simulink model "final_steady_24a"  (R2025a)
settings: Solver=ode15s  StartTime=0.0  StopTime=14000  RelTol=1e-3
undefined symbols (not defined in the file): bp_er, bp_mf, bp_speed, Cp_rad, epsilon, ETAT_table, m_ratio_bp, PR_table, speed_bp, table_eff, table_mf, theta
(part 1 of 2)
settings Model: Creator=HeY  LastModifiedBy=ikunsredemptionmac
settings DataIOCC: InitialState=xfinal  SaveFinalState=on  SaveOperatingPoint=on

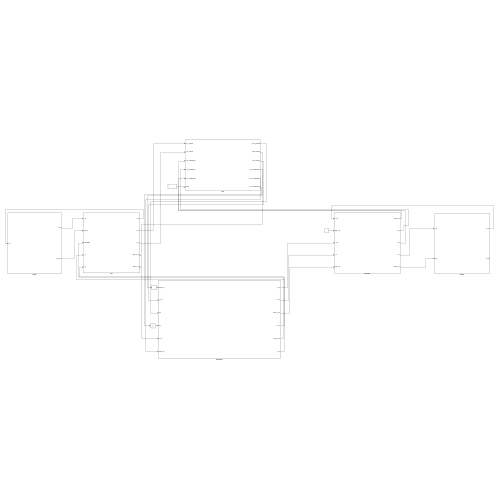
[thumbnail: Simulink's stored preview of the top-level diagram]
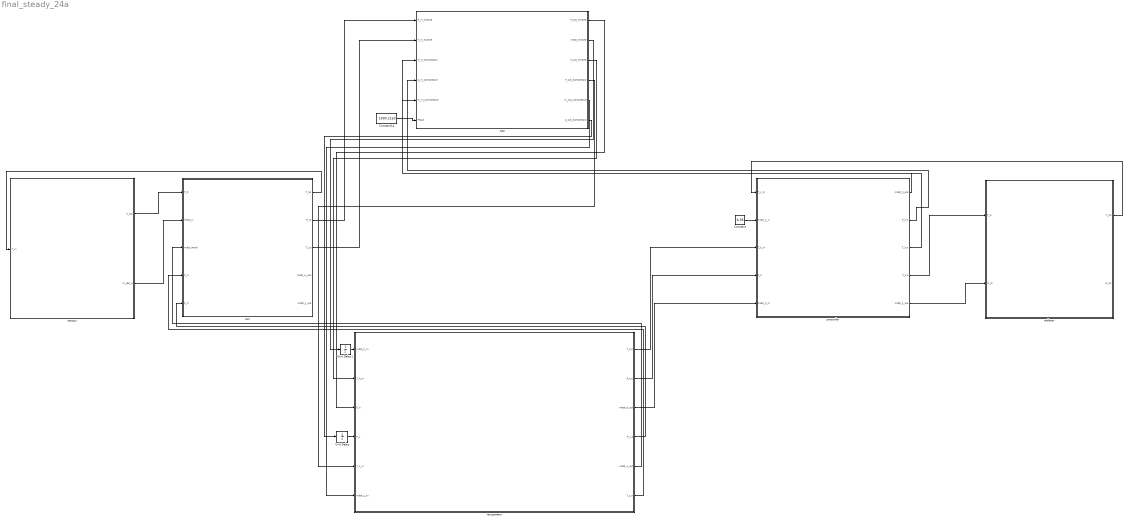
== system final_steady_24a ==
  Constant : Constant  Value=6.95
  Constant14 : Constant  Value=1000.21e3
  IHX : Subsystem
  TAC : Subsystem
  Unit Delay : UnitDelay  InitialCondition=1.551e6  SampleTime=-1  HasFrameUpgradeWarning=on
  Unit Delay1 : UnitDelay  InitialCondition=11.982029  SampleTime=-1  HasFrameUpgradeWarning=on
  precooler : Subsystem
  reactor : Subsystem
  recuperator : Subsystem
  rediator : Subsystem
  wires:
  reactor/1(T_out) -> IHX/1(T_hi)
  IHX/1(T_ho) -> reactor/1(T_in)
  reactor/2(m_dot_Li) -> IHX/2(mdot_Li)
  recuperator/6(T_c,o) -> IHX/4(T_ci)
  recuperator/4(P_c,o) -> IHX/5(P_ci)
  IHX/2(P_co) -> TAC/1(P_in_Turbine)
  IHX/3(T_co) -> TAC/2(T_in_Turbine)
  recuperator/5(mdot_c_out) -> IHX/3(mdot_HeXe)
  recuperator/3(mdot_h_out) -> precooler/5(mdot_h_in)
  recuperator/2(P_h,o) -> precooler/4(P_h)
  recuperator/1(T_h,o) -> precooler/3(T_h_in)
  Constant/1 -> precooler/2(mdot_c_in)
  precooler/3(T_h,o) -> TAC/3(T_in_Compressor)
  precooler/4(T_c,o) -> rediator/1(T_hi)
  precooler/5(mdot_c_out) -> rediator/2(m_hi)
  rediator/1(T_ho) -> precooler/1(T_c_in)
  precooler/1(mdot_h_out) -> TAC/5(m_in_Compressor)
  precooler/2(P_h,o) -> TAC/4(p_in_Compressor)
  Unit Delay/1 -> recuperator/4(P_c)
  TAC/2(mdot_Turbine) -> Unit Delay1/1
  TAC/3(T_out_Turbine) -> recuperator/2(T_h_in)
  TAC/4(T_out_Compressor) -> recuperator/5(T_c_in)
  TAC/5(m_out_Compressor) -> recuperator/6(mdot_c_in)
  TAC/6(p_out_Compressor) -> Unit Delay/1
  Constant14/1 -> TAC/6(Pload)
  TAC/1(P_out_Turbine) -> recuperator/3(P_h)
  Unit Delay1/1 -> recuperator/1(mdot_h_in)

== system final_steady_24a/IHX ==
  T_hi : Inport
  mdot_Li : Inport  Port=2
  mdot_HeXe : Inport  Port=3
  T_ci : Inport  Port=4
  P_ci : Inport  Port=5
  IHX_region_1 : Subsystem
  IHX_region_2 : Subsystem
  Scope : Scope
      settings: ActiveDisplayYMinimum=1527.0598  ActiveDisplayYMaximum=1529.6517
  Scope1 : Scope
      settings: ActiveDisplayYMinimum=1413.1189  ActiveDisplayYMaximum=1443.3824
  T_ho : Outport
  P_co : Outport  Port=2
  T_co : Outport  Port=3
  mdot_Li_out : Outport  Port=4
  mdot_c_out : Outport  Port=5
  wires:
  mdot_Li/1 -> IHX_region_1/3(mdot_Li_in)
  P_ci/1 -> IHX_region_1/2(P_HeXe_in)
  IHX_region_1/4(mdot_HeXe_out) -> mdot_c_out/1
  IHX_region_1/1(T_Li_out) -> IHX_region_2/1(T_Li_in)
  IHX_region_1/5(T_HeXe_out) -> Scope/1, T_co/1
  IHX_region_1/2(P_HeXe_out) -> IHX_region_2/2(P_HeXe_in)
  IHX_region_2/2(P_HeXe_out) -> P_co/1
  T_hi/1 -> IHX_region_1/1(T_Li_in)
  mdot_HeXe/1 -> IHX_region_2/4(mdot_HeXe_in)
  IHX_region_2/3(mdot_Li_out) -> mdot_Li_out/1
  IHX_region_2/1(T_Li_out) -> Scope1/1, T_ho/1
  IHX_region_2/4(mdot_HeXe_out) -> IHX_region_1/4(mdot_HeXe_in)
  IHX_region_2/5(T_HeXe_out) -> IHX_region_1/5(T_HeXe_in)
  T_ci/1 -> IHX_region_2/5(T_HeXe_in)
  IHX_region_1/3(mdot_Li_out) -> IHX_region_2/3(mdot_Li_in)

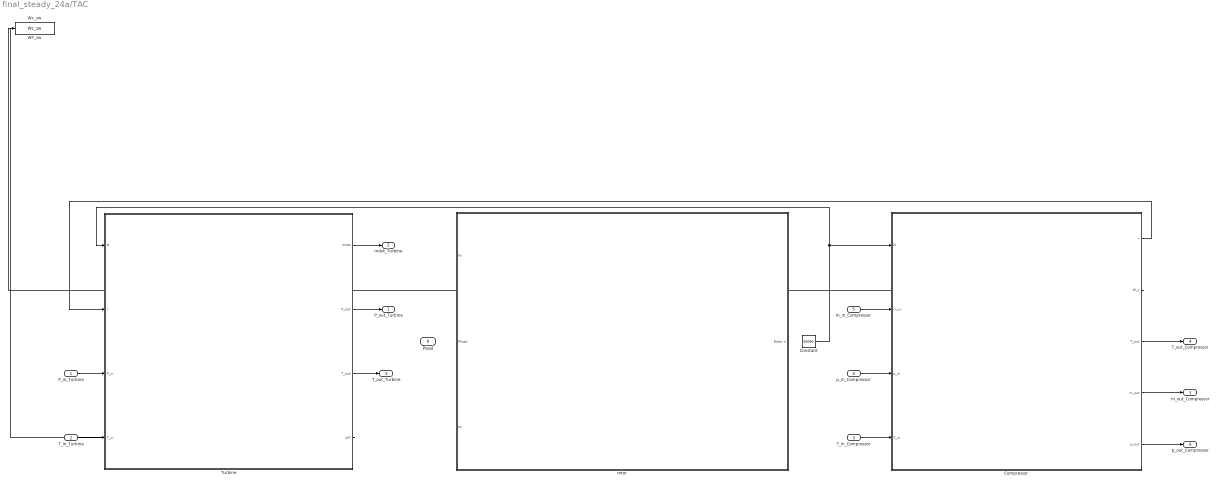
== system final_steady_24a/TAC ==
  P_in_Turbine : Inport
  T_in_Turbine : Inport  Port=2
  T_in_Compressor : Inport  Port=3
  p_in_Compressor : Inport  Port=4
  m_in_Compressor : Inport  Port=5
  Pload : Inport  Port=6
  Compressor : Subsystem
  Constant : Constant  Value=55090
  Turbine : Subsystem
  WT_sw : ToWorkspace  VariableName=WT_sw  SaveFormat=Timeseries  SampleTime=-1
  Wc_sw : ToWorkspace  VariableName=Wc_sw  SaveFormat=Timeseries  SampleTime=-1
  rotor : Subsystem
  P_out_Turbine : Outport
  mdot_Turbine : Outport  Port=2
  T_out_Turbine : Outport  Port=3
  T_out_Compressor : Outport  Port=4
  m_out_Compressor : Outport  Port=5
  p_out_Compressor : Outport  Port=6
  wires:
  Compressor/1(r) -> Turbine/2(r)
  P_in_Turbine/1 -> Turbine/3(P_in)
  T_in_Turbine/1 -> Turbine/4(T_in)
  Turbine/1(mdot) -> mdot_Turbine/1
  Turbine/2(P_out) -> P_out_Turbine/1
  Turbine/3(T_out) -> T_out_Turbine/1
  m_in_Compressor/1 -> Compressor/2(m_in)
  p_in_Compressor/1 -> Compressor/3(p_in)
  T_in_Compressor/1 -> Compressor/4(T_in)
  Compressor/3(T_out) -> T_out_Compressor/1
  Compressor/4(m_out) -> m_out_Compressor/1
  Compressor/5(p_out) -> p_out_Compressor/1
  Constant/1 -> Turbine/1(N), Compressor/1(N)
  Turbine/4(WT) -> WT_sw/1
  Compressor/2(W_c) -> Wc_sw/1

== system final_steady_24a/precooler ==
  T_c_in : Inport
  mdot_c_in : Inport  Port=2
  T_h_in : Inport  Port=3
  P_h : Inport  Port=4
  mdot_h_in : Inport  Port=5
  Scope1 : Scope
      settings: ActiveDisplayYMinimum=380.7971  ActiveDisplayYMaximum=621.9029
  precooler_1 : Subsystem
  precooler_2 : Subsystem
  mdot_h_out : Outport
  P_h,o : Outport  Port=2
  T_h,o : Outport  Port=3
  T_c,o : Outport  Port=4
  mdot_c_out : Outport  Port=5
  wires:
  precooler_1/5(T_c,o) -> T_c,o/1
  mdot_c_in/1 -> precooler_2/4(mdot_c_in)
  P_h/1 -> precooler_1/2(P_h)
  precooler_1/2(P_h,o) -> precooler_2/2(P_h)
  precooler_1/4(mdot_c_out) -> mdot_c_out/1
  precooler_2/5(T_c,o) -> precooler_1/5(T_c_in)
  precooler_1/3(mdot_h_out) -> precooler_2/3(mdot_h_in)
  precooler_1/1(T_h,o) -> precooler_2/1(T_h_in)
  mdot_h_in/1 -> precooler_1/3(mdot_h_in)
  precooler_2/2(P_h,o) -> P_h,o/1
  T_h_in/1 -> precooler_1/1(T_h_in)
  precooler_2/4(mdot_c_out) -> precooler_1/4(mdot_c_in)
  T_c_in/1 -> precooler_2/5(T_c_in)
  precooler_2/3(mdot_h_out) -> mdot_h_out/1
  precooler_2/1(T_h,o) -> Scope1/1, T_h,o/1

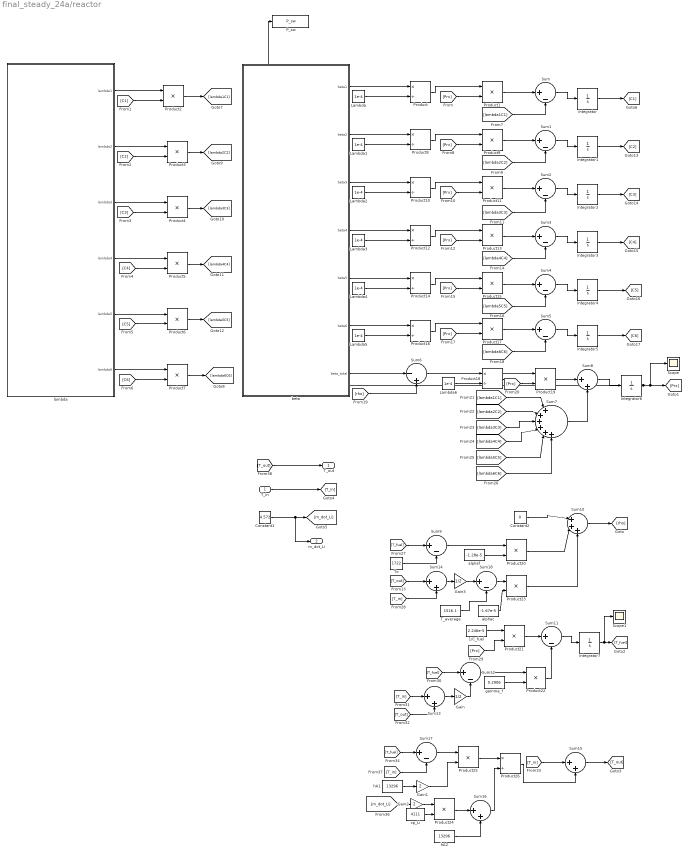
== system final_steady_24a/reactor ==
  T_in : Inport
  1/C_fuel : Constant  Value=2.246e-5
  Constant1 : Constant  Value=4.572
  Constant2 : Constant  Value=0
  Gain : Gain  Gain=1/2
  Gain1 : Gain  Gain=2
  Gain2 : Gain  Gain=2
  Gain3 : Gain  Gain=1/2
  Integrator : Integrator  InitialCondition=509563538.35378009
  Integrator1 : Integrator  InitialCondition=1144297134.5374382
  Integrator2 : Integrator  InitialCondition=278405927.94625711
  Integrator3 : Integrator  InitialCondition=222870449.79609099
  Integrator4 : Integrator  InitialCondition=15570422.720039152
  Integrator5 : Integrator  InitialCondition=1144144.4343794831
  Integrator6 : Integrator  InitialCondition=2660960.9141046703
  Integrator7 : Integrator  InitialCondition=1721.8648882133552
  Lambda{,1..6} (7 alike) : Constant  Value=1e-4
  P_sw : ToWorkspace  VariableName=P_sw  SaveFormat=Timeseries  SampleTime=-1
  Product{,8,10,12,14,16,18,26} (8 alike) : Product  Inputs=*/
  Product{1..7,9,11,13,15,17,19..25} (19 alike) : Product
  Scope : Scope
      settings: ActiveDisplayYMinimum=-1  ActiveDisplayYMaximum=1  DataLoggingVariableName=ScopeData2
  Scope1 : Scope
      settings: ActiveDisplayYMinimum=-1  ActiveDisplayYMaximum=1  DataLoggingVariableName=ScopeData3
  Sum{,1..5,9,11..12,17..18} (11 alike) : Sum  Inputs=|+-
  Sum10 : Sum  Inputs=|+++
  Sum{8,13..16} (5 alike) : Sum  Inputs=|++
  Sum6 : Sum  Inputs=|-+
  Sum7 : Sum  Inputs=|++++++
  T_average : Constant  Value=1516.1
  To : Constant  Value=1722
  alphac : Constant  Value=-1.67e-5
  alphaf : Constant  Value=-1.28e-5
  beta : Subsystem
  cp_Li : Constant  Value=4111
  gamma_f : Constant  Value=0.2906
  hA1 : Constant  Value=13296
  hA2 : Constant  Value=13296
  lambda : Subsystem
  T_out : Outport
  m_dot_Li : Outport  Port=2
  wires:
  Lambda/1 -> Product/2
  beta/1(beta1) -> Product/1
  Product/1 -> Product1/1
  [Prx] -> Product1/2
  Product1/1 -> Sum/1
  [C1] -> Product2/2
  lambda/1(lambda1) -> Product2/1
  lambda/2(lambda2) -> Product3/1
  [C2] -> Product3/2
  lambda/3(lambda3) -> Product4/1
  lambda/4(lambda4) -> Product5/1
  lambda/5(lambda5) -> Product6/1
  lambda/6(lambda6) -> Product7/1
  [C6] -> Product7/2
  [C5] -> Product6/2
  [C4] -> Product5/2
  [C3] -> Product4/2
  Product2/1 -> [lambda1C1]
  Product3/1 -> [lambda2C2]
  Product7/1 -> [lambda6C6]
  Product6/1 -> [lambda5C5]
  Product5/1 -> [lambda4C4]
  Product4/1 -> [lambda3C3]
  [lambda1C1] -> Sum/2
  Sum/1 -> Integrator/1
  Integrator/1 -> [C1]
  Integrator1/1 -> [C2]
  Sum1/1 -> Integrator1/1
  [lambda2C2] -> Sum1/2
  Product9/1 -> Sum1/1
  [Prx] -> Product9/2
  Product8/1 -> Product9/1
  beta/2(beta2) -> Product8/1
  Lambda1/1 -> Product8/2
  Lambda2/1 -> Product10/2
  beta/3(beta3) -> Product10/1
  Product10/1 -> Product11/1
  [Prx] -> Product11/2
  Product11/1 -> Sum2/1
  [lambda3C3] -> Sum2/2
  Sum2/1 -> Integrator2/1
  Integrator2/1 -> [C3]
  Integrator3/1 -> [C4]
  Sum3/1 -> Integrator3/1
  [lambda4C4] -> Sum3/2
  Product13/1 -> Sum3/1
  [Prx] -> Product13/2
  Product12/1 -> Product13/1
  Lambda3/1 -> Product12/2
  beta/4(beta4) -> Product12/1
  beta/5(beta5) -> Product14/1
  Lambda4/1 -> Product14/2
  Product14/1 -> Product15/1
  [Prx] -> Product15/2
  Product15/1 -> Sum4/1
  [lambda5C5] -> Sum4/2
  Sum4/1 -> Integrator4/1
  Integrator4/1 -> [C5]
  Integrator5/1 -> [C6]
  Sum5/1 -> Integrator5/1
  [lambda6C6] -> Sum5/2
  Product17/1 -> Sum5/1
  [Prx] -> Product17/2
  Product16/1 -> Product17/1
  Lambda5/1 -> Product16/2
  beta/6(beta6) -> Product16/1
  beta/7(beta_total) -> Sum6/1
  [rho] -> Sum6/2
  Sum6/1 -> Product18/1
  Lambda6/1 -> Product18/2
  Product18/1 -> Product19/1
  [Prx] -> Product19/2
  [lambda1C1] -> Sum7/1
  [lambda2C2] -> Sum7/2
  [lambda3C3] -> Sum7/3
  [lambda4C4] -> Sum7/4
  [lambda5C5] -> Sum7/5
  [lambda6C6] -> Sum7/6
  Sum7/1 -> Sum8/2
  Product19/1 -> Sum8/1
  Sum8/1 -> Integrator6/1
  Integrator6/1 -> Scope/1, [Prx], P_sw/1
  [T_fuel] -> Sum9/1
  To/1 -> Sum9/2
  Sum9/1 -> Product20/1
  alphaf/1 -> Product20/2
  Product20/1 -> Sum10/2
  Constant2/1 -> Sum10/1
  Sum10/1 -> [rho]
  1/C_fuel/1 -> Product21/1
  [Prx] -> Product21/2
  Product21/1 -> Sum11/1
  [T_fuel] -> Sum12/1
  [T_in] -> Sum13/1
  [T_out] -> Sum13/2
  Sum13/1 -> Gain/1
  Gain/1 -> Sum12/2
  Sum12/1 -> Product22/1
  gamma_f/1 -> Product22/2
  Product22/1 -> Sum11/2
  Sum11/1 -> Integrator7/1
  Integrator7/1 -> Scope1/1, [T_fuel]
  T_in/1 -> [T_in]
  Constant1/1 -> m_dot_Li/1, [m_dot_Li]
  [T_in] -> Sum15/1
  hA1/1 -> Gain1/1
  [m_dot_Li] -> Gain2/1
  Gain2/1 -> Product24/1
  cp_Li/1 -> Product24/2
  Product24/1 -> Sum16/1
  hA2/1 -> Sum16/2
  [T_fuel] -> Sum17/1
  [T_in] -> Sum17/2
  Sum17/1 -> Product25/1
  Gain1/1 -> Product25/2
  Product25/1 -> Product26/1
  Sum16/1 -> Product26/2
  Product26/1 -> Sum15/2
  Sum15/1 -> [T_out]
  [T_out] -> T_out/1
  Product23/1 -> Sum10/3
  alphac/1 -> Product23/2
  [T_out] -> Sum14/1
  [T_in] -> Sum14/2
  Sum14/1 -> Gain3/1
  Gain3/1 -> Sum18/1
  Sum18/1 -> Product23/1
  T_average/1 -> Sum18/2

== system final_steady_24a/recuperator ==
  mdot_h_in : Inport  OutDataTypeStr=double  Unit=kg/s  PortDimensions=1  Interpolate=off
  T_h_in : Inport  Port=2  OutDataTypeStr=double  Unit=K  PortDimensions=1  Interpolate=off
  P_h : Inport  Port=3  OutDataTypeStr=double  Unit=Pa  PortDimensions=1  Interpolate=off
  P_c : Inport  Port=4  OutDataTypeStr=double  Unit=Pa  PortDimensions=1  Interpolate=off
  T_c_in : Inport  Port=5  OutDataTypeStr=double  Unit=K  PortDimensions=1  Interpolate=off
  mdot_c_in : Inport  Port=6  OutDataTypeStr=double  Unit=kg/s  PortDimensions=1  Interpolate=off
  MannRegion_1 : Subsystem
  MannRegion_2 : Subsystem
  T_h,o : Outport  OutDataTypeStr=double  Unit=K  PortDimensions=1
  P_h,o : Outport  Port=2  OutDataTypeStr=double  Unit=Pa  PortDimensions=1
  mdot_h_out : Outport  Port=3  OutDataTypeStr=double  Unit=kg/s  PortDimensions=1
  P_c,o : Outport  Port=4  OutDataTypeStr=double  Unit=Pa  PortDimensions=1
  mdot_c_out : Outport  Port=5  OutDataTypeStr=double  Unit=kg/s  PortDimensions=1
  T_c,o : Outport  Port=6  OutDataTypeStr=double  Unit=K  PortDimensions=1
  wires:
  MannRegion_1/1(mdot_h_out) -> MannRegion_2/1(mdot_h_in)
  MannRegion_2/4(mdot_c_out) -> MannRegion_1/4(mdot_c_in)
  MannRegion_1/3(T_h,o) -> MannRegion_2/3(T_h_in)
  T_h_in/1 -> MannRegion_1/1(T_h_in)
  P_h/1 -> MannRegion_1/3(P_h)
  MannRegion_2/6(P_c,o) -> MannRegion_1/6(P_c)
  MannRegion_1/4(mdot_c_out) -> mdot_c_out/1
  MannRegion_1/6(P_c,o) -> P_c,o/1
  MannRegion_1/2(P_h,o) -> MannRegion_2/2(P_h)
  MannRegion_1/5(T_c,o) -> T_c,o/1
  mdot_h_in/1 -> MannRegion_1/2(mdot_h_in)
  P_c/1 -> MannRegion_2/6(P_c)
  T_c_in/1 -> MannRegion_2/5(T_c_in)
  mdot_c_in/1 -> MannRegion_2/4(mdot_c_in)
  MannRegion_2/2(P_h,o) -> P_h,o/1
  MannRegion_2/3(T_h,o) -> T_h,o/1
  MannRegion_2/1(mdot_h_out) -> mdot_h_out/1
  MannRegion_2/5(T_c,o) -> MannRegion_1/5(T_c_in)

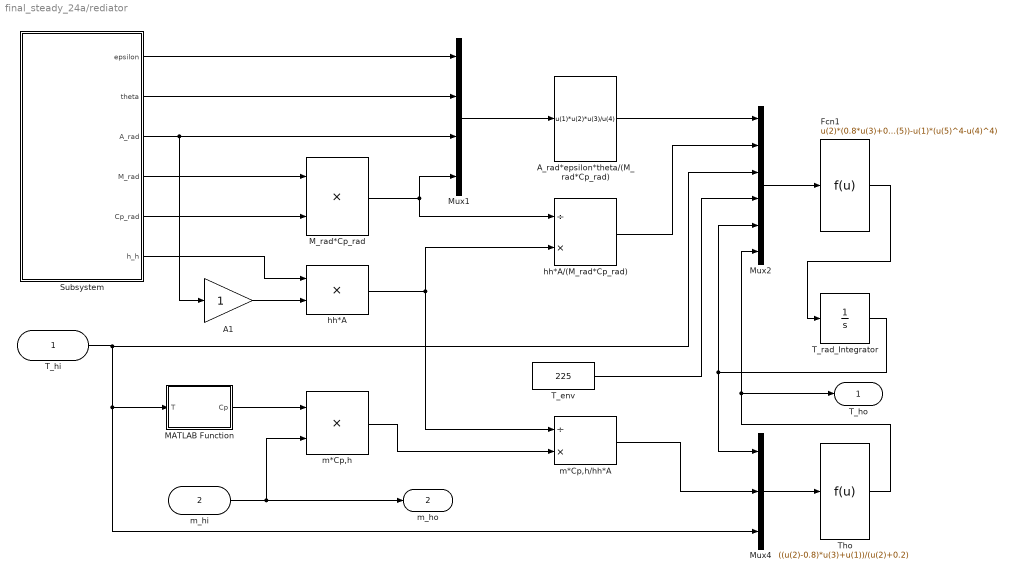
== system final_steady_24a/rediator ==
  T_hi : Inport
  m_hi : Inport  Port=2
  A1 : Gain
  A_rad*epsilon*theta/(M_rad*Cp_rad) : Fcn  Expr=u(1)*u(2)*u(3)/u(4)
  Fcn1 : Fcn  Expr=u(2)*(0.8*u(3)+0.2*u(6)-u(5))-u(1)*(u(5)^4-u(4)^4)
  MATLAB Function : MATLAB Function  TreatAsAtomicUnit=on
  M_rad*Cp_rad : Product
  Mux1 : Mux
  Mux2 : Mux  Inputs=6
  Mux4 : Mux  Inputs=3
  Subsystem : Subsystem
  T_env : Constant  Value=225
  T_rad_Integrator : Integrator  InitialCondition=416.60796744255316
  Tho : Fcn  Expr=((u(2)-0.8)*u(3)+u(1))/(u(2)+0.2)
  hh*A : Product
  hh*A/(M_rad*Cp_rad) : Product  Inputs=/*
  m*Cp,h : Product
  m*Cp,h/hh*A : Product  Inputs=/*
  T_ho : Outport
  m_ho : Outport  Port=2
  wires:
  Subsystem/5(Cp_rad) -> M_rad*Cp_rad/2
  hh*A/(M_rad*Cp_rad)/1 -> Mux2/2
  Mux4/1 -> Tho/1
  A_rad*epsilon*theta/(M_rad*Cp_rad)/1 -> Mux2/1
  Fcn1/1 -> T_rad_Integrator/1
  T_env/1 -> Mux2/4
  T_rad_Integrator/1 -> Mux4/1, Mux2/5
  M_rad*Cp_rad/1 -> hh*A/(M_rad*Cp_rad)/1, Mux1/4
  m_hi/1 -> m*Cp,h/2, m_ho/1
  m*Cp,h/1 -> m*Cp,h/hh*A/2
  T_hi/1 -> MATLAB Function/1(T), Mux4/3, Mux2/3
  MATLAB Function/1(Cp) -> m*Cp,h/1
  Subsystem/1(epsilon) -> Mux1/1
  Subsystem/4(M_rad) -> M_rad*Cp_rad/1
  Subsystem/3(A_rad) -> A1/1, Mux1/3
  Subsystem/2(theta) -> Mux1/2
  hh*A/1 -> hh*A/(M_rad*Cp_rad)/2, m*Cp,h/hh*A/1
  Mux2/1 -> Fcn1/1
  Tho/1 -> T_ho/1, Mux2/6
  Mux1/1 -> A_rad*epsilon*theta/(M_rad*Cp_rad)/1
  A1/1 -> hh*A/2
  Subsystem/6(h_h) -> hh*A/1
  m*Cp,h/hh*A/1 -> Mux4/2

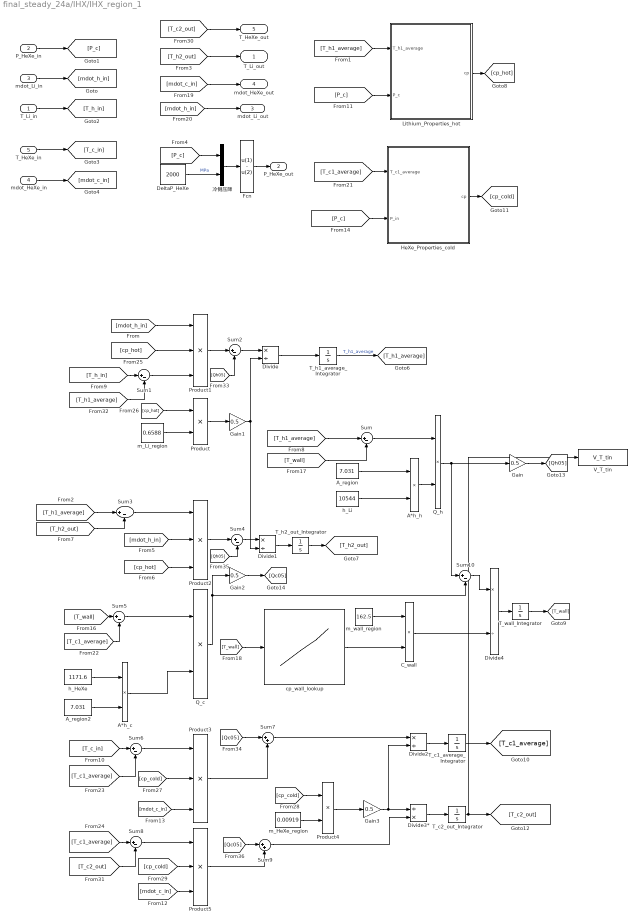
== system final_steady_24a/IHX/IHX_region_1 ==
  T_Li_in : Inport
  P_HeXe_in : Inport  Port=2
  mdot_Li_in : Inport  Port=3
  mdot_HeXe_in : Inport  Port=4
  T_HeXe_in : Inport  Port=5
  A*h_c : Product
  A*h_h : Product
  A_region : Constant  Value=7.031
  A_region2 : Constant  Value=7.031
  C_wall : Product
  DeltaP_HeXe : Constant  Value=2000
  Divide{,1..2,4} (4 alike) : Product  Inputs=*/
  Divide3* : Product  Inputs=/*
  Fcn : Fcn  Expr=u(1) - u(2)
  Gain{,1..3} (4 alike) : Gain  Gain=0.5
  HeXe_Properties_cold : MATLAB Function  TreatAsAtomicUnit=on
  Lithium_Properties_hot : MATLAB Function  TreatAsAtomicUnit=on
  Product : Product
  Product{1..3,5} (4 alike) : Product  Inputs=3
  Product4 : Product
  Q_c : Product
  Q_h : Product
  Sum{,1..6,8,10} (9 alike) : Sum  Inputs=|+-
  Sum7 : Sum  Inputs=|++
  Sum9 : Sum  Inputs=|++
  T_c1_average_Integrator : Integrator  InitialCondition=1458.2400006378589
  T_c2_out_Integrator : Integrator  InitialCondition=1522.8762873625776
  T_h1_average_Integrator : Integrator  InitialCondition=1566.8123914550606
  T_h2_out_Integrator : Integrator  InitialCondition=1544.6784341826062
  T_wall_Integrator : Integrator  InitialCondition=1555.9547816852855
  V_T_tin : ToWorkspace  VariableName=V_T_tin  SaveFormat=Timeseries  SampleTime=-1
  cp_wall_lookup : Lookup_n-D  NumberOfTableDimensions=1  BreakpointsForDimension1=[293.15, 373.15, 473.15, 573.15,673.15, 773.15, 873.15, 973.15,1073.15, 1173.15, 1273.15, 1366.48,1473.15,1573.15,1600]  Table=[419, 440, 465, 490,515, 536, 561, 586,611, 636, 662,682.4,709.6,734.1,740.7]  InternalRulePriority=Speed  RndMeth=Simplest
  h_HeXe : Constant  Value=1171.6
  h_Li : Constant  Value=10544
  m_HeXe_region : Constant  Value=0.00919
  m_Li_region : Constant  Value=0.6588
  m_wall_region : Constant  Value=162.5
  冷侧压降 : Mux  Inputs=2
  T_Li_out : Outport
  P_HeXe_out : Outport  Port=2
  mdot_Li_out : Outport  Port=3
  mdot_HeXe_out : Outport  Port=4
  T_HeXe_out : Outport  Port=5
  wires:
  mdot_HeXe_in/1 -> [mdot_c_in]
  mdot_Li_in/1 -> [mdot_h_in]
  T_h1_average_Integrator/1 -> [T_h1_average]  "T_h1_average"
  T_wall_Integrator/1 -> [T_wall]
  A_region/1 -> A*h_h/1
  h_Li/1 -> A*h_h/2
  A*h_h/1 -> Q_h/2
  T_Li_in/1 -> [T_h_in]
  Sum1/1 -> Product1/3
  Lithium_Properties_hot/1(cp) -> [cp_hot]
  Q_h/1 -> Gain/1, Sum10/1
  Product1/1 -> Sum2/1
  Gain/1 -> [Qh05]
  m_Li_region/1 -> Product/2
  Product/1 -> Gain1/1
  Sum2/1 -> Divide/1
  Gain1/1 -> Divide/2, Divide1/2
  Divide/1 -> T_h1_average_Integrator/1
  T_h2_out_Integrator/1 -> [T_h2_out]
  Sum3/1 -> Product2/1
  Product2/1 -> Sum4/1
  Sum4/1 -> Divide1/1
  Divide1/1 -> T_h2_out_Integrator/1
  T_c1_average_Integrator/1 -> [T_c1_average]
  h_HeXe/1 -> A*h_c/1
  A*h_c/1 -> Q_c/2
  Sum5/1 -> Q_c/1
  T_HeXe_in/1 -> [T_c_in]
  HeXe_Properties_cold/1(cp) -> [cp_cold]
  Q_c/1 -> Gain2/1, Sum10/2
  Gain2/1 -> [Qc05]
  Product3/1 -> Sum7/2
  m_HeXe_region/1 -> Product4/2
  Sum7/1 -> Divide2/1
  Gain3/1 -> Divide2/2, Divide3*/1
  Divide2/1 -> T_c1_average_Integrator/1
  T_c2_out_Integrator/1 -> [T_c2_out], V_T_tin/1
  Sum8/1 -> Product5/1
  Product5/1 -> Sum9/2
  Sum9/1 -> Divide3*/2
  Divide3*/1 -> T_c2_out_Integrator/1
  m_wall_region/1 -> C_wall/1
  C_wall/1 -> Divide4/2
  Sum10/1 -> Divide4/1
  Divide4/1 -> T_wall_Integrator/1
  Sum6/1 -> Product3/1
  P_HeXe_in/1 -> [P_c]
  cp_wall_lookup/1 -> C_wall/2
  DeltaP_HeXe/1 -> 冷侧压降/2  "MPa"
  Fcn/1 -> P_HeXe_out/1
  冷侧压降/1 -> Fcn/1
  [mdot_h_in] -> Product1/1
  [T_h1_average] -> Lithium_Properties_hot/1(T_h1_average)
  [T_h1_average] -> Sum3/1
  [T_h2_out] -> T_Li_out/1
  [P_c] -> 冷侧压降/1
  [mdot_h_in] -> Product2/2
  [cp_hot] -> Product2/3
  [T_h2_out] -> Sum3/2
  [T_h1_average] -> Sum/1
  [T_h_in] -> Sum1/1
  [T_c_in] -> Sum6/1
  [P_c] -> Lithium_Properties_hot/2(P_c)
  [mdot_c_in] -> Product5/3
  [mdot_c_in] -> Product3/3
  [T_wall] -> Sum5/1
  [T_wall] -> Sum/2
  [T_wall] -> cp_wall_lookup/1
  A_region2/1 -> A*h_c/2
  Sum/1 -> Q_h/1
  [mdot_c_in] -> mdot_HeXe_out/1
  [mdot_h_in] -> mdot_Li_out/1
  [T_c1_average] -> HeXe_Properties_cold/1(T_c1_average)
  [T_c1_average] -> Sum5/2
  [T_c1_average] -> Sum6/2
  [T_c1_average] -> Sum8/1
  [cp_hot] -> Product1/2
  [cp_hot] -> Product/1
  [cp_cold] -> Product3/2
  [cp_cold] -> Product4/1
  [cp_cold] -> Product5/2
  [T_c2_out] -> T_HeXe_out/1
  [T_c2_out] -> Sum8/2
  [T_h1_average] -> Sum1/2
  Product4/1 -> Gain3/1
  [Qh05] -> Sum2/2
  [Qh05] -> Sum4/2
  [Qc05] -> Sum7/1
  [Qc05] -> Sum9/1
  [P_c] -> HeXe_Properties_cold/2(P_in)

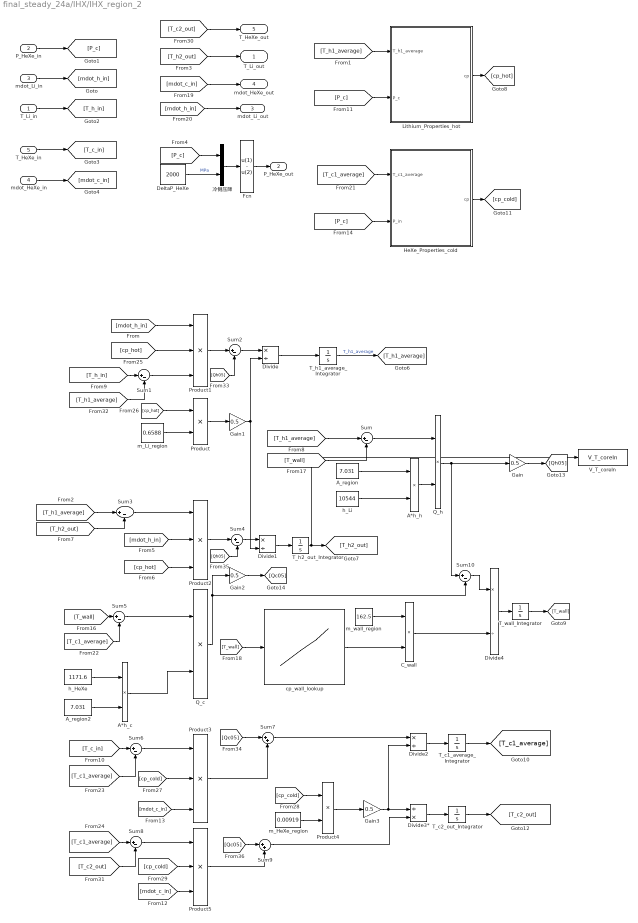
== system final_steady_24a/IHX/IHX_region_2 ==
  T_Li_in : Inport
  P_HeXe_in : Inport  Port=2
  mdot_Li_in : Inport  Port=3
  mdot_HeXe_in : Inport  Port=4
  T_HeXe_in : Inport  Port=5
  A*h_c : Product
  A*h_h : Product
  A_region : Constant  Value=7.031
  A_region2 : Constant  Value=7.031
  C_wall : Product
  DeltaP_HeXe : Constant  Value=2000
  Divide{,1..2,4} (4 alike) : Product  Inputs=*/
  Divide3* : Product  Inputs=/*
  Fcn : Fcn  Expr=u(1) - u(2)
  Gain{,1..3} (4 alike) : Gain  Gain=0.5
  HeXe_Properties_cold : MATLAB Function  TreatAsAtomicUnit=on
  Lithium_Properties_hot : MATLAB Function  TreatAsAtomicUnit=on
  Product : Product
  Product{1..3,5} (4 alike) : Product  Inputs=3
  Product4 : Product
  Q_c : Product
  Q_h : Product
  Sum{,1..6,8,10} (9 alike) : Sum  Inputs=|+-
  Sum7 : Sum  Inputs=|++
  Sum9 : Sum  Inputs=|++
  T_c1_average_Integrator : Integrator  InitialCondition=1245.8184669844006
  T_c2_out_Integrator : Integrator  InitialCondition=1393.6037139151003
  T_h1_average_Integrator : Integrator  InitialCondition=1494.0696022025936
  T_h2_out_Integrator : Integrator  InitialCondition=1443.4607702226581
  T_wall_Integrator : Integrator  InitialCondition=1469.2436410947309
  V_T_coreIn : ToWorkspace  VariableName=V_T_coreIn  SaveFormat=Timeseries  SampleTime=-1
  cp_wall_lookup : Lookup_n-D  NumberOfTableDimensions=1  BreakpointsForDimension1=[293.15, 373.15, 473.15, 573.15,673.15, 773.15, 873.15, 973.15,1073.15, 1173.15, 1273.15, 1366.48,1473.15,1573.15,1600]  Table=[419, 440, 465, 490,515, 536, 561, 586,611, 636, 662,682.4,709.6,734.1,740.7]  InternalRulePriority=Speed  RndMeth=Simplest
  h_HeXe : Constant  Value=1171.6
  h_Li : Constant  Value=10544
  m_HeXe_region : Constant  Value=0.00919
  m_Li_region : Constant  Value=0.6588
  m_wall_region : Constant  Value=162.5
  冷侧压降 : Mux  Inputs=2
  T_Li_out : Outport
  P_HeXe_out : Outport  Port=2
  mdot_Li_out : Outport  Port=3
  mdot_HeXe_out : Outport  Port=4
  T_HeXe_out : Outport  Port=5
  wires:
  mdot_HeXe_in/1 -> [mdot_c_in]
  mdot_Li_in/1 -> [mdot_h_in]
  T_h1_average_Integrator/1 -> [T_h1_average]  "T_h1_average"
  T_wall_Integrator/1 -> [T_wall]
  A_region/1 -> A*h_h/1
  h_Li/1 -> A*h_h/2
  A*h_h/1 -> Q_h/2
  T_Li_in/1 -> [T_h_in]
  Sum1/1 -> Product1/3
  Lithium_Properties_hot/1(cp) -> [cp_hot]
  Q_h/1 -> Gain/1, Sum10/1
  Product1/1 -> Sum2/1
  Gain/1 -> [Qh05]
  m_Li_region/1 -> Product/2
  Product/1 -> Gain1/1
  Sum2/1 -> Divide/1
  Gain1/1 -> Divide/2, Divide1/2
  Divide/1 -> T_h1_average_Integrator/1
  T_h2_out_Integrator/1 -> [T_h2_out], V_T_coreIn/1
  Sum3/1 -> Product2/1
  Product2/1 -> Sum4/1
  Sum4/1 -> Divide1/1
  Divide1/1 -> T_h2_out_Integrator/1
  T_c1_average_Integrator/1 -> [T_c1_average]
  h_HeXe/1 -> A*h_c/1
  A*h_c/1 -> Q_c/2
  Sum5/1 -> Q_c/1
  T_HeXe_in/1 -> [T_c_in]
  Q_c/1 -> Gain2/1, Sum10/2
  Gain2/1 -> [Qc05]
  Product3/1 -> Sum7/2
  m_HeXe_region/1 -> Product4/2
  Sum7/1 -> Divide2/1
  Gain3/1 -> Divide2/2, Divide3*/1
  Divide2/1 -> T_c1_average_Integrator/1
  T_c2_out_Integrator/1 -> [T_c2_out]
  Sum8/1 -> Product5/1
  Product5/1 -> Sum9/2
  Sum9/1 -> Divide3*/2
  Divide3*/1 -> T_c2_out_Integrator/1
  m_wall_region/1 -> C_wall/1
  C_wall/1 -> Divide4/2
  Sum10/1 -> Divide4/1
  Divide4/1 -> T_wall_Integrator/1
  Sum6/1 -> Product3/1
  P_HeXe_in/1 -> [P_c]
  cp_wall_lookup/1 -> C_wall/2
  DeltaP_HeXe/1 -> 冷侧压降/2  "MPa"
  Fcn/1 -> P_HeXe_out/1
  冷侧压降/1 -> Fcn/1
  [mdot_h_in] -> Product1/1
  [T_h1_average] -> Lithium_Properties_hot/1(T_h1_average)
  [T_h1_average] -> Sum3/1
  [T_h2_out] -> T_Li_out/1
  [P_c] -> 冷侧压降/1
  [mdot_h_in] -> Product2/2
  [cp_hot] -> Product2/3
  [T_h2_out] -> Sum3/2
  [T_h1_average] -> Sum/1
  [T_h_in] -> Sum1/1
  [T_c_in] -> Sum6/1
  [P_c] -> Lithium_Properties_hot/2(P_c)
  [mdot_c_in] -> Product5/3
  [mdot_c_in] -> Product3/3
  [T_wall] -> Sum5/1
  [T_wall] -> Sum/2
  [T_wall] -> cp_wall_lookup/1
  A_region2/1 -> A*h_c/2
  Sum/1 -> Q_h/1
  [mdot_c_in] -> mdot_HeXe_out/1
  [mdot_h_in] -> mdot_Li_out/1
  [T_c1_average] -> Sum5/2
  [T_c1_average] -> Sum6/2
  [T_c1_average] -> Sum8/1
  [cp_hot] -> Product1/2
  [cp_hot] -> Product/1
  [cp_cold] -> Product3/2
  [cp_cold] -> Product4/1
  [cp_cold] -> Product5/2
  [T_c2_out] -> T_HeXe_out/1
  [T_c2_out] -> Sum8/2
  [T_h1_average] -> Sum1/2
  Product4/1 -> Gain3/1
  [Qh05] -> Sum2/2
  [Qh05] -> Sum4/2
  [Qc05] -> Sum7/1
  [Qc05] -> Sum9/1
  [T_c1_average] -> HeXe_Properties_cold/1(T_c1_average)
  [P_c] -> HeXe_Properties_cold/2(P_in)
  HeXe_Properties_cold/1(cp) -> [cp_cold]

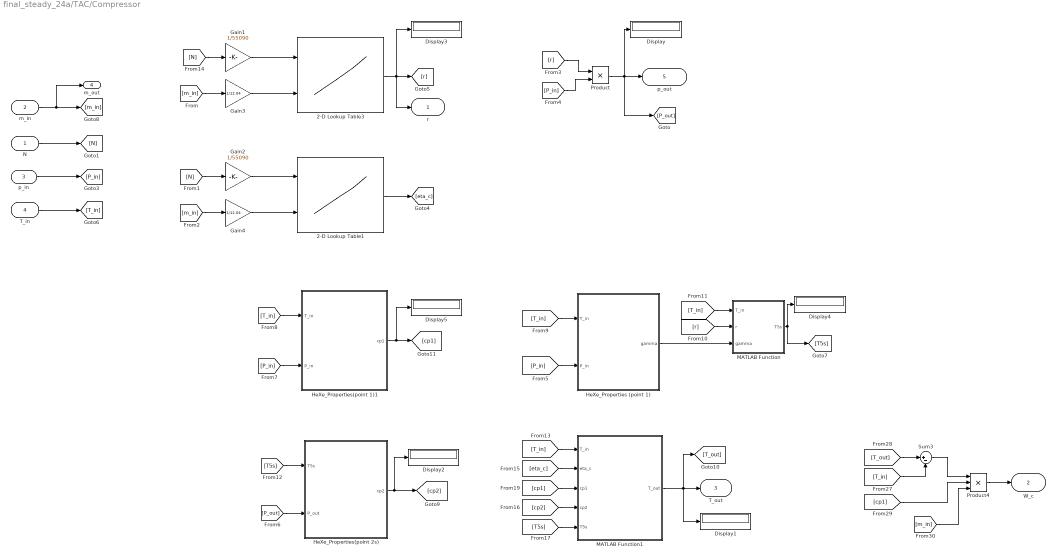
== system final_steady_24a/TAC/Compressor ==
  N : Inport
  m_in : Inport  Port=2
  p_in : Inport  Port=3
  T_in : Inport  Port=4
  2-D Lookup Table1 : Lookup_n-D  BreakpointsForDimension1=speed_bp  BreakpointsForDimension2=m_ratio_bp  Table=ETAT_table  ExtrapMethod=Clip  InternalRulePriority=Speed  RndMeth=Simplest
      settings: InputPortMap=u0,u1
  2-D Lookup Table3 : Lookup_n-D  BreakpointsForDimension1=speed_bp  BreakpointsForDimension2=m_ratio_bp  Table=PR_table  ExtrapMethod=Clip  InternalRulePriority=Speed  RndMeth=Simplest
      settings: InputPortMap=u0,u1
  Display{,1..5} (6 alike) : Display
  Gain1 : Gain  Gain=1/55090
  Gain2 : Gain  Gain=1/55090
  Gain3 : Gain  Gain=1/12.04
  Gain4 : Gain  Gain=1/12.04
  HeXe_Properties (point 1) : MATLAB Function  TreatAsAtomicUnit=on
  HeXe_Properties(point 1)1 : MATLAB Function  TreatAsAtomicUnit=on
  HeXe_Properties(point 2s) : MATLAB Function  TreatAsAtomicUnit=on
  MATLAB Function : MATLAB Function  TreatAsAtomicUnit=on
  MATLAB Function1 : MATLAB Function  TreatAsAtomicUnit=on
  Product : Product
  Product4 : Product  Inputs=3
  Sum3 : Sum  Inputs=|+-
  r : Outport
  W_c : Outport  Port=2
  T_out : Outport  Port=3
  m_out : Outport  Port=4
  p_out : Outport  Port=5
  wires:
  [N] -> Gain1/1
  Gain2/1 -> 2-D Lookup Table1/1
  [N] -> Gain2/1
  2-D Lookup Table3/1 -> r/1, Display3/1, [r]
  [m_in] -> Gain4/1
  m_in/1 -> m_out/1, [m_in]
  2-D Lookup Table1/1 -> [eta_c]
  Gain1/1 -> 2-D Lookup Table3/1
  Gain3/1 -> 2-D Lookup Table3/2
  Gain4/1 -> 2-D Lookup Table1/2
  N/1 -> [N]
  [m_in] -> Gain3/1
  T_in/1 -> [T_in]
  p_in/1 -> [P_in]
  [P_in] -> Product/2
  [r] -> Product/1
  Product/1 -> Display/1, [P_out], p_out/1
  [cp1] -> Product4/2
  Sum3/1 -> Product4/1
  [m_in] -> Product4/3
  MATLAB Function1/1(T_out) -> [T_out], Display1/1, T_out/1
  Product4/1 -> W_c/1
  [T_in] -> HeXe_Properties(point 1)1/1(T_in)
  [P_in] -> HeXe_Properties(point 1)1/2(P_in)
  HeXe_Properties(point 1)1/1(cp1) -> [cp1], Display5/1
  MATLAB Function/1(T5s) -> [T5s], Display4/1
  [T_in] -> HeXe_Properties (point 1)/1(T_in)
  [P_in] -> HeXe_Properties (point 1)/2(P_in)
  [r] -> MATLAB Function/2(r)
  [T_in] -> MATLAB Function/1(T_in)
  HeXe_Properties(point 2s)/1(cp2) -> [cp2], Display2/1
  [T5s] -> HeXe_Properties(point 2s)/1(T5s)
  [P_out] -> HeXe_Properties(point 2s)/2(P_out)
  [T5s] -> MATLAB Function1/5(T5s)
  [T_in] -> MATLAB Function1/1(T_in)
  [cp2] -> MATLAB Function1/4(cp2)
  [eta_c] -> MATLAB Function1/2(eta_c)
  [cp1] -> MATLAB Function1/3(cp1)
  HeXe_Properties (point 1)/1(gamma) -> MATLAB Function/3(gamma)
  [T_in] -> Sum3/2
  [T_out] -> Sum3/1

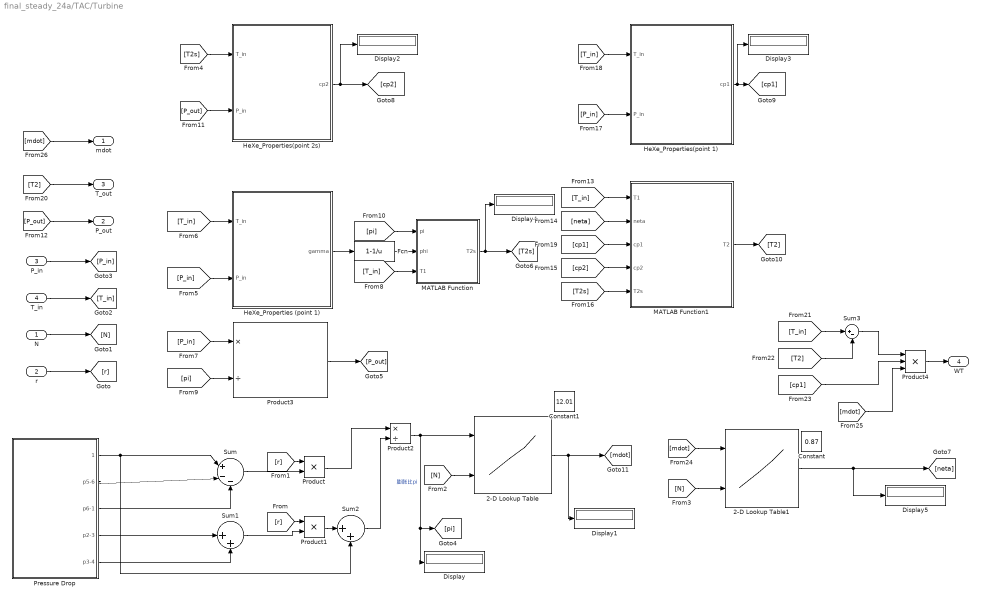
== system final_steady_24a/TAC/Turbine ==
  N : Inport
  r : Inport  Port=2
  P_in : Inport  Port=3
  T_in : Inport  Port=4
  2-D Lookup Table : Lookup_n-D  BreakpointsForDimension1=bp_er  BreakpointsForDimension2=bp_speed  Table=table_mf  InternalRulePriority=Speed  RndMeth=Simplest
      settings: InputPortMap=u0,u1
  2-D Lookup Table1 : Lookup_n-D  BreakpointsForDimension1=bp_mf  BreakpointsForDimension2=bp_speed  Table=table_eff  InternalRulePriority=Speed  RndMeth=Simplest
      settings: InputPortMap=u0,u1
  Constant : Constant  Value=0.87
  Constant1 : Constant  Value=12.01
  Display{,1..5} (6 alike) : Display
  Fcn : Fcn  Expr=1-1/u
  HeXe_Properties (point 1) : MATLAB Function  TreatAsAtomicUnit=on
  HeXe_Properties(point 1) : MATLAB Function  TreatAsAtomicUnit=on
  HeXe_Properties(point 2s) : MATLAB Function  TreatAsAtomicUnit=on
  MATLAB Function : MATLAB Function  TreatAsAtomicUnit=on
  MATLAB Function1 : MATLAB Function  TreatAsAtomicUnit=on
  Pressure Drop : Subsystem
  Product : Product
  Product1 : Product
  Product2 : Product  Inputs=*/
  Product3 : Product  Inputs=*/
  Product4 : Product  Inputs=3
  Sum : Sum  Inputs=|+--
  Sum1 : Sum  Inputs=|++
  Sum2 : Sum  Inputs=|++
  Sum3 : Sum  Inputs=|+-
  mdot : Outport
  P_out : Outport  Port=2
  T_out : Outport  Port=3
  WT : Outport  Port=4
  wires:
  Fcn/1 -> MATLAB Function/2(phi)
  Product4/1 -> WT/1
  Product3/1 -> [P_out]
  [P_out] -> HeXe_Properties(point 2s)/2(P_in)
  [cp1] -> Product4/2
  [pi] -> MATLAB Function/1(pi)
  [T2s] -> HeXe_Properties(point 2s)/1(T_in)
  MATLAB Function1/1(T2) -> [T2]
  N/1 -> [N]
  [T2] -> Sum3/2
  [T_in] -> MATLAB Function/3(T1)
  [N] -> 2-D Lookup Table/2
  T_in/1 -> [T_in]
  Sum2/1 -> Product2/2
  2-D Lookup Table1/1 -> [neta], Display5/1
  HeXe_Properties (point 1)/1(gamma) -> Fcn/1
  Product1/1 -> Sum2/1
  [T2] -> T_out/1
  Sum/1 -> Product/2
  r/1 -> [r]
  Product/1 -> Product2/1
  Pressure Drop/2(p5-6) -> Sum/2
  [r] -> Product/1
  [pi] -> Product3/2
  [cp1] -> MATLAB Function1/3(cp1)
  [r] -> Product1/1
  [T_in] -> MATLAB Function1/1(T1)
  Sum3/1 -> Product4/1
  [T2s] -> MATLAB Function1/5(T2s)
  Pressure Drop/4(p2-3) -> Sum1/1
  [T_in] -> HeXe_Properties (point 1)/1(T_in)
  [P_in] -> HeXe_Properties (point 1)/2(P_in)
  Pressure Drop/5(p3-4) -> Sum1/2
  HeXe_Properties(point 2s)/1(cp2) -> [cp2], Display2/1
  Pressure Drop/3(p6-1) -> Sum/3
  [cp2] -> MATLAB Function1/4(cp2)
  MATLAB Function/1(T2s) -> Display4/1, [T2s]
  [neta] -> MATLAB Function1/2(neta)
  Sum1/1 -> Product1/2
  [P_out] -> P_out/1
  [T_in] -> Sum3/1
  Pressure Drop/1(1) -> Sum2/2, Sum/1
  HeXe_Properties(point 1)/1(cp1) -> Display3/1, [cp1]
  Product2/1 -> 2-D Lookup Table/1, Display/1, [pi]  "膨胀比pi"
  [T_in] -> HeXe_Properties(point 1)/1(T_in)
  P_in/1 -> [P_in]
  [P_in] -> HeXe_Properties(point 1)/2(P_in)
  [N] -> 2-D Lookup Table1/2
  [P_in] -> Product3/1
  2-D Lookup Table/1 -> Display1/1, [mdot]
  [mdot] -> 2-D Lookup Table1/1
  [mdot] -> Product4/3
  [mdot] -> mdot/1

== system final_steady_24a/TAC/rotor ==
  Pc : Inport
  Pload : Inport  Port=2
  Pt : Inport  Port=3
  Coeff : Constant  Value=900/((pi^2)*0.5)
  Floor : Rounding
  N_rpm_Integrator : Integrator  InitialCondition=55090
  Product : Product  Inputs=**/
  Sum : Sum  Inputs=|+--
  Rotor n : Outport
  wires:
  N_rpm_Integrator/1 -> Product/3, Rotor n/1
  Coeff/1 -> Product/1
  Pt/1 -> Sum/1
  Pc/1 -> Sum/2
  Pload/1 -> Sum/3
  Sum/1 -> Floor/1
  Floor/1 -> Product/2

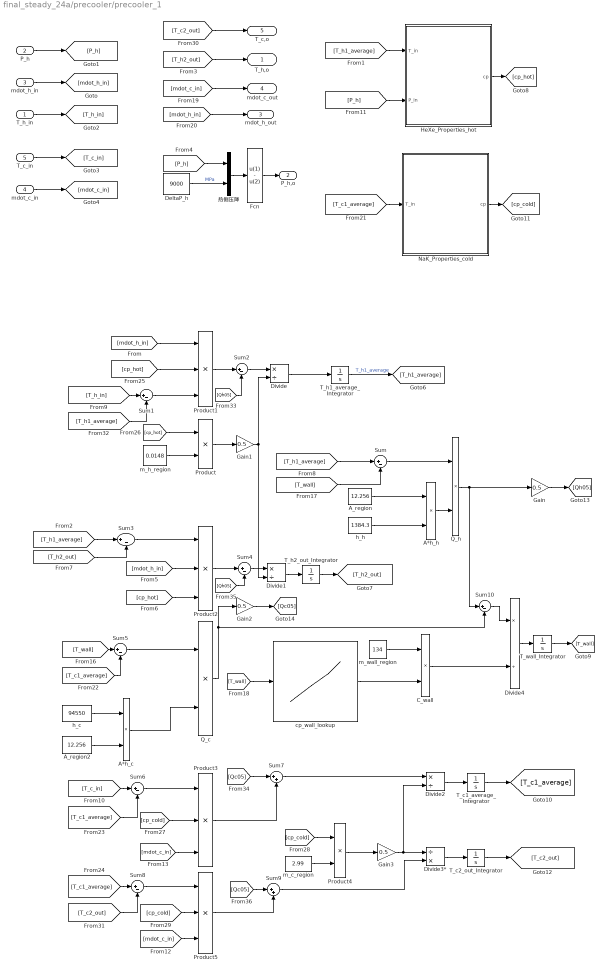
== system final_steady_24a/precooler/precooler_1 ==
  T_h_in : Inport
  P_h : Inport  Port=2
  mdot_h_in : Inport  Port=3
  mdot_c_in : Inport  Port=4
  T_c_in : Inport  Port=5
  A*h_c : Product
  A*h_h : Product
  A_region : Constant  Value=12.256
  A_region2 : Constant  Value=12.256
  C_wall : Product
  DeltaP_h : Constant  Value=9000
  Divide{,1..2,4} (4 alike) : Product  Inputs=*/
  Divide3* : Product  Inputs=/*
  Fcn : Fcn  Expr=u(1) - u(2)
  Gain{,1..3} (4 alike) : Gain  Gain=0.5
  HeXe_Properties_hot : MATLAB Function  TreatAsAtomicUnit=on
  NaK_Properties_cold : MATLAB Function  TreatAsAtomicUnit=on
  Product : Product
  Product{1..3,5} (4 alike) : Product  Inputs=3
  Product4 : Product
  Q_c : Product
  Q_h : Product
  Sum{,1..6,8,10} (9 alike) : Sum  Inputs=|+-
  Sum7 : Sum  Inputs=|++
  Sum9 : Sum  Inputs=|++
  T_c1_average_Integrator : Integrator  InitialCondition=545.7329915378557
  T_c2_out_Integrator : Integrator  InitialCondition=611.57676479754946
  T_h1_average_Integrator : Integrator  InitialCondition=594.86709308142633
  T_h2_out_Integrator : Integrator  InitialCondition=528.91021598735142
  T_wall_Integrator : Integrator  InitialCondition=546.44198026309198
  cp_wall_lookup : Lookup_n-D  NumberOfTableDimensions=1  BreakpointsForDimension1=[300, 325, 350, 375, 400, 425, 450, 475, 500, 525, 550, 575, 600, 625, 650, 675, 700, 725, 750, 775, 800, 825, 850, 875, 900, 925, 950, 975, 1000]  Table=[469.94, 478.26, 485.85, 492.85, 499.36, 505.49, 511.28, 516.80, 522.08, 527.16, 532.06, 536.82, 541.44, 545.94, 550.35, 554.66, 558.88, 563.04, 567.13, 571.16, 575.13, 579.06, 582.94, 586.78, 590.58, 594.35, 598.08, 601.79, 605.47]  InternalRulePriority=Speed  RndMeth=Simplest
  h_c : Constant  Value=94550
  h_h : Constant  Value=1384.3
  m_c_region : Constant  Value=2.99
  m_h_region : Constant  Value=0.0148
  m_wall_region : Constant  Value=134
  热侧压降 : Mux  Inputs=2
  T_h,o : Outport
  P_h,o : Outport  Port=2
  mdot_h_out : Outport  Port=3
  mdot_c_out : Outport  Port=4
  T_c,o : Outport  Port=5
  wires:
  mdot_c_in/1 -> [mdot_c_in]
  mdot_h_in/1 -> [mdot_h_in]
  T_h1_average_Integrator/1 -> [T_h1_average]  "T_h1_average"
  T_wall_Integrator/1 -> [T_wall]
  A_region/1 -> A*h_h/1
  h_h/1 -> A*h_h/2
  A*h_h/1 -> Q_h/2
  T_h_in/1 -> [T_h_in]
  Sum1/1 -> Product1/3
  HeXe_Properties_hot/1(cp) -> [cp_hot]
  Q_h/1 -> Gain/1, Sum10/1
  Product1/1 -> Sum2/1
  Gain/1 -> [Qh05]
  m_h_region/1 -> Product/2
  Product/1 -> Gain1/1
  Sum2/1 -> Divide/1
  Gain1/1 -> Divide/2, Divide1/2
  Divide/1 -> T_h1_average_Integrator/1
  T_h2_out_Integrator/1 -> [T_h2_out]
  Sum3/1 -> Product2/1
  Product2/1 -> Sum4/1
  Sum4/1 -> Divide1/1
  Divide1/1 -> T_h2_out_Integrator/1
  T_c1_average_Integrator/1 -> [T_c1_average]
  h_c/1 -> A*h_c/1
  A*h_c/1 -> Q_c/2
  Sum5/1 -> Q_c/1
  T_c_in/1 -> [T_c_in]
  NaK_Properties_cold/1(cp) -> [cp_cold]
  Q_c/1 -> Gain2/1, Sum10/2
  Gain2/1 -> [Qc05]
  Product3/1 -> Sum7/2
  m_c_region/1 -> Product4/2
  Sum7/1 -> Divide2/1
  Gain3/1 -> Divide2/2, Divide3*/1
  Divide2/1 -> T_c1_average_Integrator/1
  T_c2_out_Integrator/1 -> [T_c2_out]
  Sum8/1 -> Product5/1
  Product5/1 -> Sum9/2
  Sum9/1 -> Divide3*/2
  Divide3*/1 -> T_c2_out_Integrator/1
  m_wall_region/1 -> C_wall/1
  C_wall/1 -> Divide4/2
  Sum10/1 -> Divide4/1
  Divide4/1 -> T_wall_Integrator/1
  Sum6/1 -> Product3/1
  P_h/1 -> [P_h]
  cp_wall_lookup/1 -> C_wall/2
  DeltaP_h/1 -> 热侧压降/2  "MPa"
  Fcn/1 -> P_h,o/1
  热侧压降/1 -> Fcn/1
  [mdot_h_in] -> Product1/1
  [T_h1_average] -> HeXe_Properties_hot/1(T_in)
  [T_h1_average] -> Sum3/1
  [T_h2_out] -> T_h,o/1
  [P_h] -> 热侧压降/1
  [mdot_h_in] -> Product2/2
  [cp_hot] -> Product2/3
  [T_h2_out] -> Sum3/2
  [T_h1_average] -> Sum/1
  [T_h_in] -> Sum1/1
  [T_c_in] -> Sum6/1
  [P_h] -> HeXe_Properties_hot/2(P_in)
  [mdot_c_in] -> Product5/3
  [mdot_c_in] -> Product3/3
  [T_wall] -> Sum5/1
  [T_wall] -> Sum/2
  [T_wall] -> cp_wall_lookup/1
  A_region2/1 -> A*h_c/2
  Sum/1 -> Q_h/1
  [mdot_c_in] -> mdot_c_out/1
  [mdot_h_in] -> mdot_h_out/1
  [T_c1_average] -> NaK_Properties_cold/1(T_in)
  [T_c1_average] -> Sum5/2
  [T_c1_average] -> Sum6/2
  [T_c1_average] -> Sum8/1
  [cp_hot] -> Product1/2
  [cp_hot] -> Product/1
  [cp_cold] -> Product3/2
  [cp_cold] -> Product4/1
  [cp_cold] -> Product5/2
  [T_c2_out] -> T_c,o/1
  [T_c2_out] -> Sum8/2
  [T_h1_average] -> Sum1/2
  Product4/1 -> Gain3/1
  [Qh05] -> Sum2/2
  [Qh05] -> Sum4/2
  [Qc05] -> Sum7/1
  [Qc05] -> Sum9/1

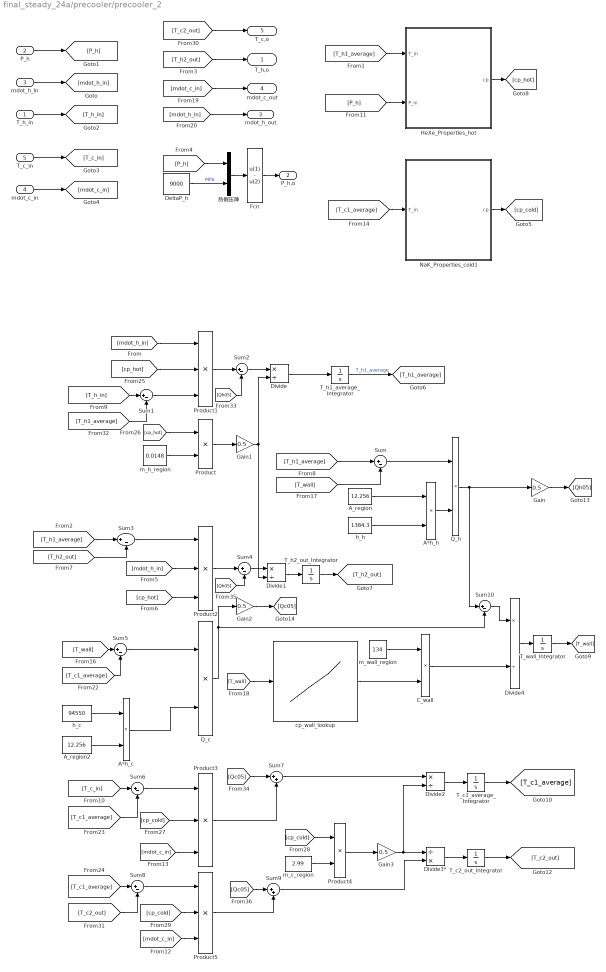
== system final_steady_24a/precooler/precooler_2 ==
  T_h_in : Inport
  P_h : Inport  Port=2
  mdot_h_in : Inport  Port=3
  mdot_c_in : Inport  Port=4
  T_c_in : Inport  Port=5
  A*h_c : Product
  A*h_h : Product
  A_region : Constant  Value=12.256
  A_region2 : Constant  Value=12.256
  C_wall : Product
  DeltaP_h : Constant  Value=9000
  Divide{,1..2,4} (4 alike) : Product  Inputs=*/
  Divide3* : Product  Inputs=/*
  Fcn : Fcn  Expr=u(1) - u(2)
  Gain{,1..3} (4 alike) : Gain  Gain=0.5
  HeXe_Properties_hot : MATLAB Function  TreatAsAtomicUnit=on
  NaK_Properties_cold1 : MATLAB Function  TreatAsAtomicUnit=on
  Product : Product
  Product{1..3,5} (4 alike) : Product  Inputs=3
  Product4 : Product
  Q_c : Product
  Q_h : Product
  Sum{,1..6,8,10} (9 alike) : Sum  Inputs=|+-
  Sum7 : Sum  Inputs=|++
  Sum9 : Sum  Inputs=|++
  T_c1_average_Integrator : Integrator  InitialCondition=418.75053506849412
  T_c2_out_Integrator : Integrator  InitialCondition=479.88921827813124
  T_h1_average_Integrator : Integrator  InitialCondition=465.7869648085188
  T_h2_out_Integrator : Integrator  InitialCondition=402.66371363139297
  T_wall_Integrator : Integrator  InitialCondition=419.42925508558875
  cp_wall_lookup : Lookup_n-D  NumberOfTableDimensions=1  BreakpointsForDimension1=[300, 325, 350, 375, 400, 425, 450, 475, 500, 525, 550, 575, 600, 625, 650, 675, 700, 725, 750, 775, 800, 825, 850, 875, 900, 925, 950, 975, 1000]  Table=[469.94, 478.26, 485.85, 492.85, 499.36, 505.49, 511.28, 516.80, 522.08, 527.16, 532.06, 536.82, 541.44, 545.94, 550.35, 554.66, 558.88, 563.04, 567.13, 571.16, 575.13, 579.06, 582.94, 586.78, 590.58, 594.35, 598.08, 601.79, 605.47]  InternalRulePriority=Speed  RndMeth=Simplest
  h_c : Constant  Value=94550
  h_h : Constant  Value=1384.3
  m_c_region : Constant  Value=2.99
  m_h_region : Constant  Value=0.0148
  m_wall_region : Constant  Value=134
  热侧压降 : Mux  Inputs=2
  T_h,o : Outport
  P_h,o : Outport  Port=2
  mdot_h_out : Outport  Port=3
  mdot_c_out : Outport  Port=4
  T_c,o : Outport  Port=5
  wires:
  mdot_c_in/1 -> [mdot_c_in]
  mdot_h_in/1 -> [mdot_h_in]
  T_h1_average_Integrator/1 -> [T_h1_average]  "T_h1_average"
  T_wall_Integrator/1 -> [T_wall]
  A_region/1 -> A*h_h/1
  h_h/1 -> A*h_h/2
  A*h_h/1 -> Q_h/2
  T_h_in/1 -> [T_h_in]
  Sum1/1 -> Product1/3
  HeXe_Properties_hot/1(cp) -> [cp_hot]
  Q_h/1 -> Gain/1, Sum10/1
  Product1/1 -> Sum2/1
  Gain/1 -> [Qh05]
  m_h_region/1 -> Product/2
  Product/1 -> Gain1/1
  Sum2/1 -> Divide/1
  Gain1/1 -> Divide/2, Divide1/2
  Divide/1 -> T_h1_average_Integrator/1
  T_h2_out_Integrator/1 -> [T_h2_out]
  Sum3/1 -> Product2/1
  Product2/1 -> Sum4/1
  Sum4/1 -> Divide1/1
  Divide1/1 -> T_h2_out_Integrator/1
  T_c1_average_Integrator/1 -> [T_c1_average]
  h_c/1 -> A*h_c/1
  A*h_c/1 -> Q_c/2
  Sum5/1 -> Q_c/1
  T_c_in/1 -> [T_c_in]
  Q_c/1 -> Gain2/1, Sum10/2
  Gain2/1 -> [Qc05]
  Product3/1 -> Sum7/2
  m_c_region/1 -> Product4/2
  Sum7/1 -> Divide2/1
  Gain3/1 -> Divide2/2, Divide3*/1
  Divide2/1 -> T_c1_average_Integrator/1
  T_c2_out_Integrator/1 -> [T_c2_out]
  Sum8/1 -> Product5/1
  Product5/1 -> Sum9/2
  Sum9/1 -> Divide3*/2
  Divide3*/1 -> T_c2_out_Integrator/1
  m_wall_region/1 -> C_wall/1
  C_wall/1 -> Divide4/2
  Sum10/1 -> Divide4/1
  Divide4/1 -> T_wall_Integrator/1
  Sum6/1 -> Product3/1
  P_h/1 -> [P_h]
  cp_wall_lookup/1 -> C_wall/2
  DeltaP_h/1 -> 热侧压降/2  "MPa"
  Fcn/1 -> P_h,o/1
  热侧压降/1 -> Fcn/1
  [mdot_h_in] -> Product1/1
  [T_h1_average] -> HeXe_Properties_hot/1(T_in)
  [T_h1_average] -> Sum3/1
  [T_h2_out] -> T_h,o/1
  [P_h] -> 热侧压降/1
  [mdot_h_in] -> Product2/2
  [cp_hot] -> Product2/3
  [T_h2_out] -> Sum3/2
  [T_h1_average] -> Sum/1
  [T_h_in] -> Sum1/1
  [T_c_in] -> Sum6/1
  [P_h] -> HeXe_Properties_hot/2(P_in)
  [mdot_c_in] -> Product5/3
  [mdot_c_in] -> Product3/3
  [T_wall] -> Sum5/1
  [T_wall] -> Sum/2
  [T_wall] -> cp_wall_lookup/1
  A_region2/1 -> A*h_c/2
  Sum/1 -> Q_h/1
  [mdot_c_in] -> mdot_c_out/1
  [mdot_h_in] -> mdot_h_out/1
  [T_c1_average] -> Sum5/2
  [T_c1_average] -> Sum6/2
  [T_c1_average] -> Sum8/1
  [cp_hot] -> Product1/2
  [cp_hot] -> Product/1
  [cp_cold] -> Product3/2
  [cp_cold] -> Product4/1
  [cp_cold] -> Product5/2
  [T_c2_out] -> T_c,o/1
  [T_c2_out] -> Sum8/2
  [T_h1_average] -> Sum1/2
  Product4/1 -> Gain3/1
  [Qh05] -> Sum2/2
  [Qh05] -> Sum4/2
  [Qc05] -> Sum7/1
  [Qc05] -> Sum9/1
  NaK_Properties_cold1/1(cp) -> [cp_cold]
  [T_c1_average] -> NaK_Properties_cold1/1(T_in)

== system final_steady_24a/reactor/beta ==
  Constant : Constant  Value=2.432e-4
  Constant1 : Constant  Value=1.3632e-3
  Constant2 : Constant  Value=1.2032e-3
  Constant3 : Constant  Value=2.6048e-3
  Constant4 : Constant  Value=8.192e-4
  Constant5 : Constant  Value=1.664e-4
  Constant6 : Constant  Value=6.4e-3
  beta1 : Outport
  beta2 : Outport  Port=2
  beta3 : Outport  Port=3
  beta4 : Outport  Port=4
  beta5 : Outport  Port=5
  beta6 : Outport  Port=6
  beta_total : Outport  Port=7
  wires:
  Constant/1 -> beta1/1
  Constant1/1 -> beta2/1
  Constant2/1 -> beta3/1
  Constant3/1 -> beta4/1
  Constant4/1 -> beta5/1
  Constant5/1 -> beta6/1
  Constant6/1 -> beta_total/1

== system final_steady_24a/reactor/lambda ==
  Constant : Constant  Value=0.0127
  Constant1 : Constant  Value=0.0317
  Constant2 : Constant  Value=0.115
  Constant3 : Constant  Value=0.311
  Constant4 : Constant  Value=1.4
  Constant5 : Constant  Value=3.87
  lambda1 : Outport
  lambda2 : Outport  Port=2
  lambda3 : Outport  Port=3
  lambda4 : Outport  Port=4
  lambda5 : Outport  Port=5
  lambda6 : Outport  Port=6
  wires:
  Constant/1 -> lambda1/1
  Constant1/1 -> lambda2/1
  Constant2/1 -> lambda3/1
  Constant3/1 -> lambda4/1
  Constant4/1 -> lambda5/1
  Constant5/1 -> lambda6/1

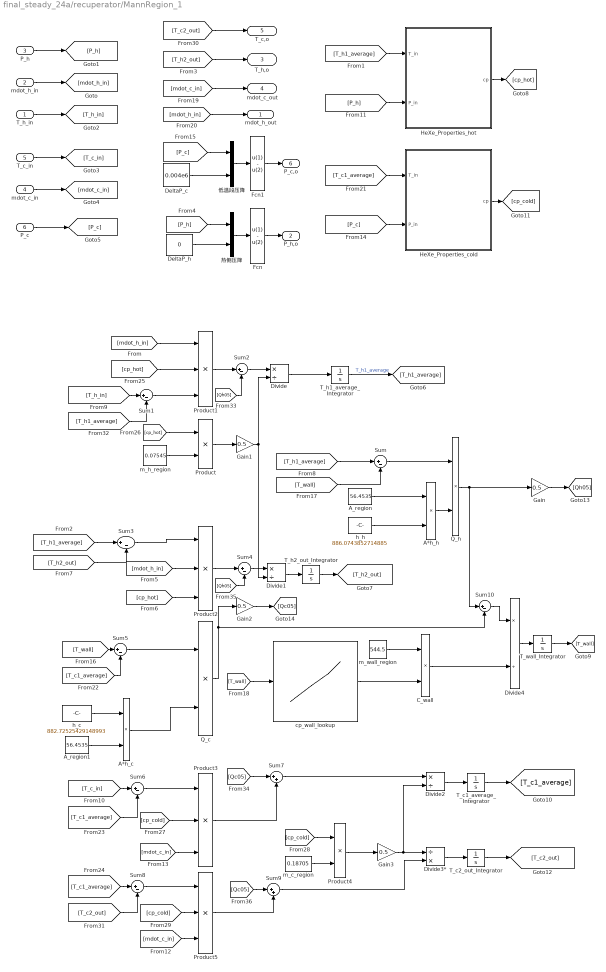
== system final_steady_24a/recuperator/MannRegion_1 ==
  T_h_in : Inport
  mdot_h_in : Inport  Port=2
  P_h : Inport  Port=3
  mdot_c_in : Inport  Port=4
  T_c_in : Inport  Port=5
  P_c : Inport  Port=6
  A*h_c : Product
  A*h_h : Product
  A_region : Constant  Value=56.4535
  A_region1 : Constant  Value=56.4535
  C_wall : Product
  DeltaP_c : Constant  Value=0.004e6
  DeltaP_h : Constant  Value=0
  Divide{,1..2,4} (4 alike) : Product  Inputs=*/
  Divide3* : Product  Inputs=/*
  Fcn : Fcn  Expr=u(1) - u(2)
  Fcn1 : Fcn  Expr=u(1) - u(2)
  Gain{,1..3} (4 alike) : Gain  Gain=0.5
  HeXe_Properties_cold : MATLAB Function  TreatAsAtomicUnit=on
  HeXe_Properties_hot : MATLAB Function  TreatAsAtomicUnit=on
  Product : Product
  Product{1..3,5} (4 alike) : Product  Inputs=3
  Product4 : Product
  Q_c : Product
  Q_h : Product
  Sum{,1..6,8,10} (9 alike) : Sum  Inputs=|+-
  Sum7 : Sum  Inputs=|++
  Sum9 : Sum  Inputs=|++
  T_c1_average_Integrator : Integrator  InitialCondition=973.10015023326082
  T_c2_out_Integrator : Integrator  InitialCondition=1098.0332200511998
  T_h1_average_Integrator : Integrator  InitialCondition=1035.4335921350307
  T_h2_out_Integrator : Integrator  InitialCondition=910.48054303365655
  T_wall_Integrator : Integrator  InitialCondition=1004.3258841003104
  cp_wall_lookup : Lookup_n-D  NumberOfTableDimensions=1  BreakpointsForDimension1=[293.15, 373.15, 473.15, 573.15, 673.15,773.15, 873.15, 973.15, 1073.15, 1173.15,1273.15]  Table=[419, 440, 465, 490, 515,536, 561, 586, 611, 636, 662]  InternalRulePriority=Speed  RndMeth=Simplest
  h_c : Constant  Value=882.72525429148993
  h_h : Constant  Value=886.0743852714885
  m_c_region : Constant  Value=0.18705
  m_h_region : Constant  Value=0.07545
  m_wall_region : Constant  Value=544.5
  低温段压降 : Mux  Inputs=2
  热侧压降 : Mux  Inputs=2
  mdot_h_out : Outport
  P_h,o : Outport  Port=2
  T_h,o : Outport  Port=3
  mdot_c_out : Outport  Port=4
  T_c,o : Outport  Port=5
  P_c,o : Outport  Port=6
  wires:
  mdot_c_in/1 -> [mdot_c_in]
  mdot_h_in/1 -> [mdot_h_in]
  T_h1_average_Integrator/1 -> [T_h1_average]  "T_h1_average"
  T_wall_Integrator/1 -> [T_wall]
  A_region/1 -> A*h_h/1
  h_h/1 -> A*h_h/2
  A*h_h/1 -> Q_h/2
  T_h_in/1 -> [T_h_in]
  Sum1/1 -> Product1/3
  HeXe_Properties_hot/1(cp) -> [cp_hot]
  Q_h/1 -> Gain/1, Sum10/1
  Product1/1 -> Sum2/1
  Gain/1 -> [Qh05]
  m_h_region/1 -> Product/2
  Product/1 -> Gain1/1
  Sum2/1 -> Divide/1
  Gain1/1 -> Divide/2, Divide1/2
  Divide/1 -> T_h1_average_Integrator/1
  T_h2_out_Integrator/1 -> [T_h2_out]
  Sum3/1 -> Product2/1
  Product2/1 -> Sum4/1
  Sum4/1 -> Divide1/1
  Divide1/1 -> T_h2_out_Integrator/1
  T_c1_average_Integrator/1 -> [T_c1_average]
  h_c/1 -> A*h_c/1
  A*h_c/1 -> Q_c/2
  Sum5/1 -> Q_c/1
  T_c_in/1 -> [T_c_in]
  HeXe_Properties_cold/1(cp) -> [cp_cold]
  Q_c/1 -> Gain2/1, Sum10/2
  Gain2/1 -> [Qc05]
  Product3/1 -> Sum7/2
  m_c_region/1 -> Product4/2
  Sum7/1 -> Divide2/1
  Gain3/1 -> Divide2/2, Divide3*/1
  Divide2/1 -> T_c1_average_Integrator/1
  T_c2_out_Integrator/1 -> [T_c2_out]
  Sum8/1 -> Product5/1
  Product5/1 -> Sum9/2
  Sum9/1 -> Divide3*/2
  Divide3*/1 -> T_c2_out_Integrator/1
  m_wall_region/1 -> C_wall/1
  C_wall/1 -> Divide4/2
  Sum10/1 -> Divide4/1
  Divide4/1 -> T_wall_Integrator/1
  Sum6/1 -> Product3/1
  P_h/1 -> [P_h]
  P_c/1 -> [P_c]
  cp_wall_lookup/1 -> C_wall/2
  DeltaP_c/1 -> 低温段压降/2
  DeltaP_h/1 -> 热侧压降/2
  Fcn/1 -> P_h,o/1
  热侧压降/1 -> Fcn/1
  低温段压降/1 -> Fcn1/1
  Fcn1/1 -> P_c,o/1
  [mdot_h_in] -> Product1/1
  [T_h1_average] -> HeXe_Properties_hot/1(T_in)
  [T_h1_average] -> Sum3/1
  [T_h2_out] -> T_h,o/1
  [P_h] -> 热侧压降/1
  [mdot_h_in] -> Product2/2
  [cp_hot] -> Product2/3
  [T_h2_out] -> Sum3/2
  [T_h1_average] -> Sum/1
  [T_h_in] -> Sum1/1
  [T_c_in] -> Sum6/1
  [P_h] -> HeXe_Properties_hot/2(P_in)
  [mdot_c_in] -> Product5/3
  [mdot_c_in] -> Product3/3
  [P_c] -> HeXe_Properties_cold/2(P_in)
  [P_c] -> 低温段压降/1
  [T_wall] -> Sum5/1
  [T_wall] -> Sum/2
  [T_wall] -> cp_wall_lookup/1
  A_region1/1 -> A*h_c/2
  Sum/1 -> Q_h/1
  [mdot_c_in] -> mdot_c_out/1
  [mdot_h_in] -> mdot_h_out/1
  [T_c1_average] -> HeXe_Properties_cold/1(T_in)
  [T_c1_average] -> Sum5/2
  [T_c1_average] -> Sum6/2
  [T_c1_average] -> Sum8/1
  [cp_hot] -> Product1/2
  [cp_hot] -> Product/1
  [cp_cold] -> Product3/2
  [cp_cold] -> Product4/1
  [cp_cold] -> Product5/2
  [T_c2_out] -> T_c,o/1
  [T_c2_out] -> Sum8/2
  [T_h1_average] -> Sum1/2
  Product4/1 -> Gain3/1
  [Qh05] -> Sum2/2
  [Qh05] -> Sum4/2
  [Qc05] -> Sum7/1
  [Qc05] -> Sum9/1

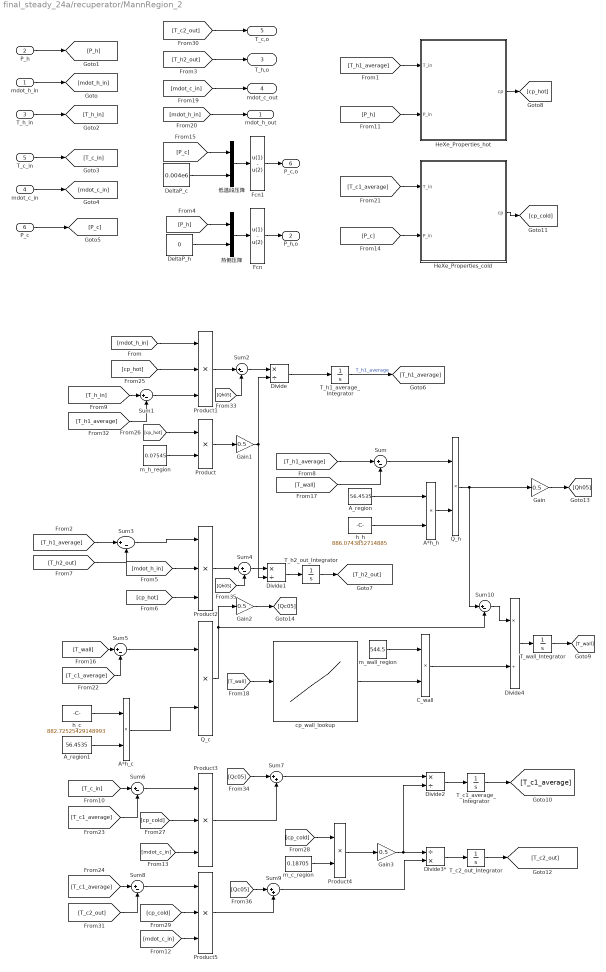
== system final_steady_24a/recuperator/MannRegion_2 ==
  mdot_h_in : Inport
  P_h : Inport  Port=2
  T_h_in : Inport  Port=3
  mdot_c_in : Inport  Port=4
  T_c_in : Inport  Port=5
  P_c : Inport  Port=6
  A*h_c : Product
  A*h_h : Product
  A_region : Constant  Value=56.4535
  A_region1 : Constant  Value=56.4535
  C_wall : Product
  DeltaP_c : Constant  Value=0.004e6
  DeltaP_h : Constant  Value=0
  Divide{,1..2,4} (4 alike) : Product  Inputs=*/
  Divide3* : Product  Inputs=/*
  Fcn : Fcn  Expr=u(1) - u(2)
  Fcn1 : Fcn  Expr=u(1) - u(2)
  Gain{,1..3} (4 alike) : Gain  Gain=0.5
  HeXe_Properties_cold : MATLAB Function  TreatAsAtomicUnit=on
  HeXe_Properties_hot : MATLAB Function  TreatAsAtomicUnit=on
  Product : Product
  Product{1..3,5} (4 alike) : Product  Inputs=3
  Product4 : Product
  Q_c : Product
  Q_h : Product
  Sum{,1..6,8,10} (9 alike) : Sum  Inputs=|+-
  Sum7 : Sum  Inputs=|++
  Sum9 : Sum  Inputs=|++
  T_c1_average_Integrator : Integrator  InitialCondition=723.37593583663499
  T_c2_out_Integrator : Integrator  InitialCondition=848.16708041554273
  T_h1_average_Integrator : Integrator  InitialCondition=785.65225660536589
  T_h2_out_Integrator : Integrator  InitialCondition=660.82397017724622
  T_wall_Integrator : Integrator  InitialCondition=754.57305466037838
  cp_wall_lookup : Lookup_n-D  NumberOfTableDimensions=1  BreakpointsForDimension1=[293.15, 373.15, 473.15, 573.15, 673.15,773.15, 873.15, 973.15, 1073.15, 1173.15,1273.15]  Table=[419, 440, 465, 490, 515,536, 561, 586, 611, 636, 662]  InternalRulePriority=Speed  RndMeth=Simplest
  h_c : Constant  Value=882.72525429148993
  h_h : Constant  Value=886.0743852714885
  m_c_region : Constant  Value=0.18705
  m_h_region : Constant  Value=0.07545
  m_wall_region : Constant  Value=544.5
  低温段压降 : Mux  Inputs=2
  热侧压降 : Mux  Inputs=2
  mdot_h_out : Outport
  P_h,o : Outport  Port=2
  T_h,o : Outport  Port=3
  mdot_c_out : Outport  Port=4
  T_c,o : Outport  Port=5
  P_c,o : Outport  Port=6
  wires:
  mdot_c_in/1 -> [mdot_c_in]
  mdot_h_in/1 -> [mdot_h_in]
  T_h1_average_Integrator/1 -> [T_h1_average]  "T_h1_average"
  T_wall_Integrator/1 -> [T_wall]
  A_region/1 -> A*h_h/1
  h_h/1 -> A*h_h/2
  A*h_h/1 -> Q_h/2
  T_h_in/1 -> [T_h_in]
  Sum1/1 -> Product1/3
  Q_h/1 -> Gain/1, Sum10/1
  Product1/1 -> Sum2/1
  Gain/1 -> [Qh05]
  m_h_region/1 -> Product/2
  Product/1 -> Gain1/1
  Sum2/1 -> Divide/1
  Gain1/1 -> Divide/2, Divide1/2
  Divide/1 -> T_h1_average_Integrator/1
  T_h2_out_Integrator/1 -> [T_h2_out]
  Sum3/1 -> Product2/1
  Product2/1 -> Sum4/1
  Sum4/1 -> Divide1/1
  Divide1/1 -> T_h2_out_Integrator/1
  T_c1_average_Integrator/1 -> [T_c1_average]
  h_c/1 -> A*h_c/1
  A*h_c/1 -> Q_c/2
  Sum5/1 -> Q_c/1
  T_c_in/1 -> [T_c_in]
  Q_c/1 -> Gain2/1, Sum10/2
  Gain2/1 -> [Qc05]
  Product3/1 -> Sum7/2
  m_c_region/1 -> Product4/2
  Sum7/1 -> Divide2/1
  Gain3/1 -> Divide2/2, Divide3*/1
  Divide2/1 -> T_c1_average_Integrator/1
  T_c2_out_Integrator/1 -> [T_c2_out]
  Sum8/1 -> Product5/1
  Product5/1 -> Sum9/2
  Sum9/1 -> Divide3*/2
  Divide3*/1 -> T_c2_out_Integrator/1
  m_wall_region/1 -> C_wall/1
  C_wall/1 -> Divide4/2
  Sum10/1 -> Divide4/1
  Divide4/1 -> T_wall_Integrator/1
  Sum6/1 -> Product3/1
  P_h/1 -> [P_h]
  P_c/1 -> [P_c]
  cp_wall_lookup/1 -> C_wall/2
  DeltaP_c/1 -> 低温段压降/2
  DeltaP_h/1 -> 热侧压降/2
  Fcn/1 -> P_h,o/1
  热侧压降/1 -> Fcn/1
  低温段压降/1 -> Fcn1/1
  Fcn1/1 -> P_c,o/1
  [mdot_h_in] -> Product1/1
  [T_h1_average] -> Sum3/1
  [T_h2_out] -> T_h,o/1
  [P_h] -> 热侧压降/1
  [mdot_h_in] -> Product2/2
  [cp_hot] -> Product2/3
  [T_h2_out] -> Sum3/2
  [T_h1_average] -> Sum/1
  [T_h_in] -> Sum1/1
  [T_c_in] -> Sum6/1
  [mdot_c_in] -> Product5/3
  [mdot_c_in] -> Product3/3
  [P_c] -> 低温段压降/1
  [T_wall] -> Sum5/1
  [T_wall] -> Sum/2
  [T_wall] -> cp_wall_lookup/1
  A_region1/1 -> A*h_c/2
  Sum/1 -> Q_h/1
  [mdot_c_in] -> mdot_c_out/1
  [mdot_h_in] -> mdot_h_out/1
  [T_c1_average] -> Sum5/2
  [T_c1_average] -> Sum6/2
  [T_c1_average] -> Sum8/1
  [cp_hot] -> Product1/2
  [cp_hot] -> Product/1
  [cp_cold] -> Product3/2
  [cp_cold] -> Product4/1
  [cp_cold] -> Product5/2
  [T_c2_out] -> T_c,o/1
  [T_c2_out] -> Sum8/2
  [T_h1_average] -> Sum1/2
  Product4/1 -> Gain3/1
  [Qh05] -> Sum2/2
  [Qh05] -> Sum4/2
  [Qc05] -> Sum7/1
  [Qc05] -> Sum9/1
  HeXe_Properties_cold/1(cp) -> [cp_cold]
  [P_h] -> HeXe_Properties_hot/2(P_in)
  [T_c1_average] -> HeXe_Properties_cold/1(T_in)
  [P_c] -> HeXe_Properties_cold/2(P_in)
  [T_h1_average] -> HeXe_Properties_hot/1(T_in)
  HeXe_Properties_hot/1(cp) -> [cp_hot]

== system final_steady_24a/rediator/Subsystem ==
  Constant : Constant  Value=epsilon
  Constant1 : Constant  Value=theta
  Constant2 : Constant  Value=1113
  Constant3 : Constant  Value=5744
  Constant4 : Constant  Value=Cp_rad
  Constant5 : Constant  Value=9.755
  epsilon : Outport
  theta : Outport  Port=2
  A_rad : Outport  Port=3
  M_rad : Outport  Port=4
  Cp_rad : Outport  Port=5
  h_h : Outport  Port=6
  wires:
  Constant3/1 -> M_rad/1
  Constant5/1 -> h_h/1
  Constant2/1 -> A_rad/1
  Constant1/1 -> theta/1
  Constant/1 -> epsilon/1
  Constant4/1 -> Cp_rad/1

== system final_steady_24a/TAC/Turbine/Pressure Drop ==
  2-3 : Constant  Value=0
  3-4 : Constant  Value=0.011605
  5-6 : Constant  Value=0.005158
  6-1 : Constant  Value=0.002579
  constant : Constant
  1 : Outport
  p5-6 : Outport  Port=2
  p6-1 : Outport  Port=3
  p2-3 : Outport  Port=4
  p3-4 : Outport  Port=5
  wires:
  5-6/1 -> p5-6/1
  3-4/1 -> p3-4/1
  constant/1 -> 1/1
  6-1/1 -> p6-1/1
  2-3/1 -> p2-3/1

== matlab function final_steady_24a/IHX/IHX_region_1/HeXe_Properties_cold ==
  data: T_c1_average input; cp output; P_in input
function cp = HeXe_Properties_cold(T_c1_average,P_in)

coder.extrinsic('HeXe_property_simulink');

cp = 0;
[cp, ~, ~, ~, ~, ~] = ...
    HeXe_property_simulink(T_c1_average, P_in);
end
